simulink library "ChimeRouterLibBtc"  (R2022b)
settings: Solver=VariableStepAuto  StartTime=0.0  StopTime=10.0  RelTol=1e-3
libraries: TuneVar x3, FeaturePath x2, HandyTextFile x1, dspindex x1, RTC x1
settings Model: Creator=kl13806  LastModifiedBy=kl13806
settings SolverCC: AlgebraicLoopSolver=TrustRegion
settings DebuggingCC: UnconnectedInputMsg=warning  UnconnectedOutputMsg=warning  UnconnectedLineMsg=warning  SFMachineParentedDataDiag=warning
settings ModelReferenceCC: EnableRefExpFcnMdlSchedulingChecks=on
settings RTWCC: DLArmComputeVersion=19.05

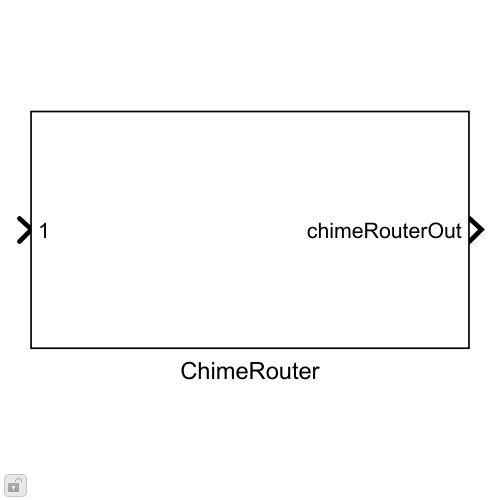
[thumbnail: Simulink's stored preview of the top-level diagram]
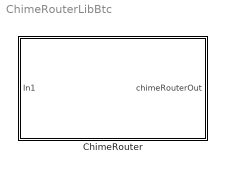
== system ChimeRouterLibBtc ==
  ChimeRouter : Subsystem  mask(Chimes ChimeRouter){Config=[]}
      mask prompts: Config "ChimeRouterConfig"
      mask init:
      | blkh=gcbh;
      | Config=BTConfig.Assert(blkh,Config);
      | 
      | Config.Validate();

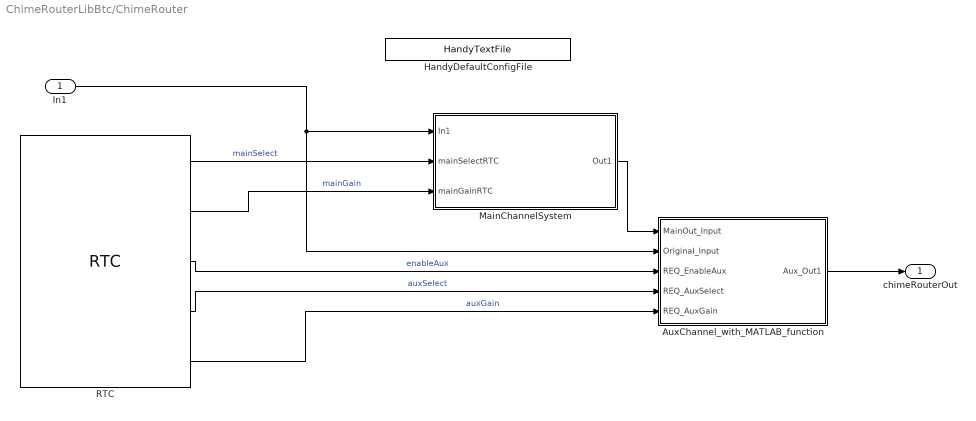
== system ChimeRouterLibBtc/ChimeRouter ==
  In1 : Inport
  AuxChannel_with_MATLAB_function : Subsystem
  HandyDefaultConfigFile : HandyTextFile/HandyTextFile  TemplateSource=Config  FileSuffix=Init  OpenDialogOnLoad=off  UseThisBlockName=off  AddGrandParentNamePrefix=off  TheDefaultText=|  ShowInLibBrowser=on
      | % $(FILENAME) Setup model parameters for each "Init" callback (e.g. update diagram)
      | sample_rate_in_hertz = 44100;
      | frame_size = 32;
      | sysin_channel_count = 2;
      settings: SourceProductName=Bose Talaria
  MainChannelSystem : Subsystem
  RTC : RTC/RTC  REQ_Priority=RTC_Mask.NormalPriority  RequestAtInit=off  EnableRequest=off  REQElemName1=MainSelect  REQElemType1=int32  REQElemWidth1=length(Config.MainSelect(:)')  REQElemInitial1=[]  REQElemName2=MainGain  REQElemType2=single  REQElemWidth2=length(Config.MainGain)  REQElemInitial2=[]  REQElemName3=EnableAux  REQElemType3=int32  REQElemWidth3=length(Config.EnableAux)  REQElemInitial3=[]  REQElemName4=AuxSelect  REQElemType4=int32  REQElemWidth4=length(Config.PAuxSelect)  REQElemInitial4=[]  REQElemName5=AuxGain  REQElemType5=single  REQElemWidth5=length(Config.PAuxGain)  REQElemInitial5=[]  REQElemType6=uint32  REQElemWidth6=1  REQElemInitial6=[]  REQElemType7=uint32  REQElemWidth7=1  REQElemInitial7=[]  REQElemType8=uint32  REQElemWidth8=1  REQElemInitial8=[]  REQElemType9=uint32  REQElemWidth9=1  REQElemInitial9=[]  REQElemType10=uint32  REQElemWidth10=1  REQElemInitial10=[]  EnableResponse=on  EnableRSP_StatusIn=off  RSPElemType1=uint32  RSPElemWidth1=1  RSPElemType2=uint32  RSPElemWidth2=1  RSPElemType3=uint32  RSPElemWidth3=1  RSPElemType4=uint32  RSPElemWidth4=1  RSPElemType5=uint32  RSPElemWidth5=1  RSPElemType6=uint32  RSPElemWidth6=1  RSPElemType7=uint32  RSPElemWidth7=1  RSPElemType8=uint32  RSPElemWidth8=1  RSPElemType9=uint32  RSPElemWidth9=1  RSPElemType10=uint32  RSPElemWidth10=1  EnableNotification=off  EnableNTF_PrepTrig=off  NTFElemType1=uint32  NTFElemWidth1=1  NTFElemType2=uint32  NTFElemWidth2=1  NTFElemType3=uint32  NTFElemWidth3=1  NTFElemType4=uint32  NTFElemWidth4=1  NTFElemType5=uint32  NTFElemWidth5=1  NTFElemType6=uint32  NTFElemWidth6=1  NTFElemType7=uint32  NTFElemWidth7=1  NTFElemType8=uint32  NTFElemWidth8=1  NTFElemType9=uint32  NTFElemWidth9=1  NTFElemType10=uint32  NTFElemWidth10=1  MaskMessageName=Set
      settings: SourceProductName=Bose Talaria
  chimeRouterOut : Outport  VectorParamsAs1DForOutWhenUnconnected=off
  wires:
  MainChannelSystem/1(Out1) -> AuxChannel_with_MATLAB_function/1(MainOut_Input)
  AuxChannel_with_MATLAB_function/1(Aux_Out1) -> chimeRouterOut/1
  In1/1 -> AuxChannel_with_MATLAB_function/2(Original_Input), MainChannelSystem/1(In1)
  RTC/3 -> AuxChannel_with_MATLAB_function/3(REQ_EnableAux)  "enableAux"
  RTC/4 -> AuxChannel_with_MATLAB_function/4(REQ_AuxSelect)  "auxSelect"
  RTC/5 -> AuxChannel_with_MATLAB_function/5(REQ_AuxGain)  "auxGain"
  RTC/1 -> MainChannelSystem/2(mainSelectRTC)  "mainSelect"
  RTC/2 -> MainChannelSystem/3(mainGainRTC)  "mainGain"

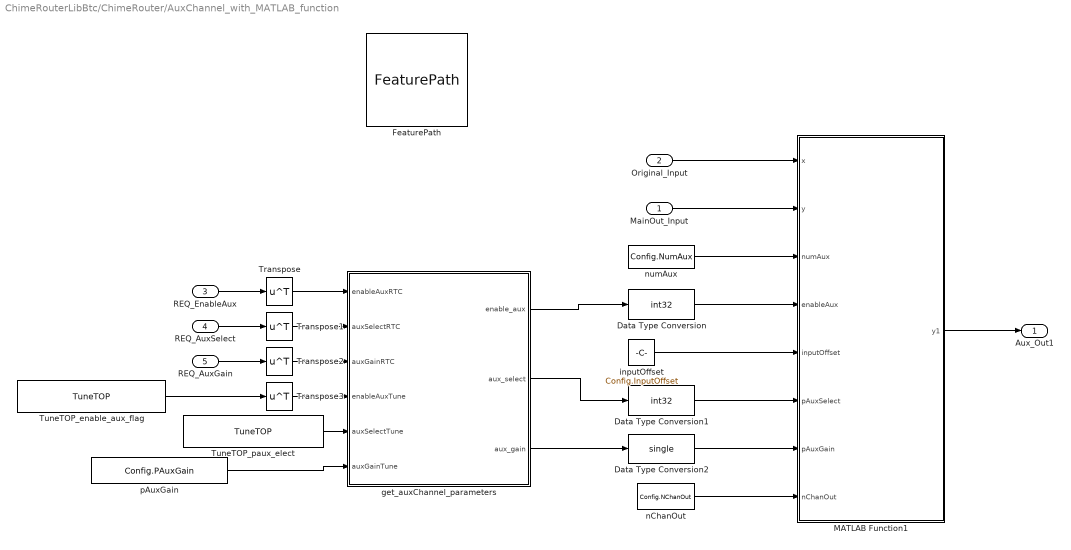
== system ChimeRouterLibBtc/ChimeRouter/AuxChannel_with_MATLAB_function ==
  MainOut_Input : Inport  PortDimensions=[Config.FrameSize Config.NChanOut]
  Original_Input : Inport  Port=2
  REQ_EnableAux : Inport  Port=3
  REQ_AuxSelect : Inport  Port=4
  REQ_AuxGain : Inport  Port=5
  Data Type Conversion : DataTypeConversion  OutDataTypeStr=int32  SaturateOnIntegerOverflow=off  RndMeth=Floor
  Data Type Conversion1 : DataTypeConversion  OutDataTypeStr=int32  SaturateOnIntegerOverflow=off  RndMeth=Floor
  Data Type Conversion2 : DataTypeConversion  OutDataTypeStr=single  SaturateOnIntegerOverflow=off  RndMeth=Floor
  FeaturePath : FeaturePath/FeaturePath  FeatureName=ASDRouterAuxChannel  IsGroup=on  GroupNumber=-1  IsModule=off  TriggerInit=[450 -186 565 -79]
      settings: SourceProductName=Bose Talaria
  MATLAB Function1 : MATLAB Function  TreatAsAtomicUnit=on
  Transpose{,1..3} (4 alike) : Math  Operator=transpose  SignedPower=on
  TuneTOP_enable_aux_flag : TuneVar/TuneTOP  TriggerInit=[50 212 220 248]  TopName=tune_top_enable_aux  TuneName=tune_top_enable_aux  DataType=int32  TunabilityNumber=1  MinValue=[]  MaxValue=[]  BankNumber=0  PreOverlay=false  PostOverlay=false  UseSameName=on  MaskValue=Config.EnableAux
      settings: SourceProductName=Bose Talaria
  TuneTOP_paux_elect : TuneVar/TuneTOP  TriggerInit=[240 252 400 288]  TopName=tune_top_paux_select  TuneName=tune_top_paux_select  DataType=int32  TunabilityNumber=1  MinValue=[]  MaxValue=[]  BankNumber=0  PreOverlay=false  PostOverlay=false  UseSameName=on  MaskValue=Config.PAuxSelect
      settings: SourceProductName=Bose Talaria
  get_auxChannel_parameters : MATLAB Function  TreatAsAtomicUnit=on
  inputOffset : Constant  Value=Config.InputOffset  OutDataTypeStr=int32
  nChanOut : Constant  Value=Config.NChanOut  OutDataTypeStr=int32
  numAux : Constant  Value=Config.NumAux  OutDataTypeStr=int32
  pAuxGain : Constant  Value=Config.PAuxGain  VectorParams1D=off  OutDataTypeStr=single
  Aux_Out1 : Outport  PortDimensions=[Config.FrameSize Config.NChanOut]  VectorParamsAs1DForOutWhenUnconnected=off
  wires:
  nChanOut/1 -> MATLAB Function1/8(nChanOut)
  REQ_EnableAux/1 -> Transpose/1
  TuneTOP_paux_elect/1 -> get_auxChannel_parameters/5(auxSelectTune)
  Transpose/1 -> get_auxChannel_parameters/1(enableAuxRTC)
  Transpose2/1 -> get_auxChannel_parameters/3(auxGainRTC)
  TuneTOP_enable_aux_flag/1 -> Transpose3/1
  inputOffset/1 -> MATLAB Function1/5(inputOffset)
  MainOut_Input/1 -> MATLAB Function1/2(y)
  MATLAB Function1/1(y1) -> Aux_Out1/1
  get_auxChannel_parameters/1(enable_aux) -> Data Type Conversion/1
  Transpose1/1 -> get_auxChannel_parameters/2(auxSelectRTC)
  REQ_AuxGain/1 -> Transpose2/1
  get_auxChannel_parameters/2(aux_select) -> Data Type Conversion1/1
  Data Type Conversion2/1 -> MATLAB Function1/7(pAuxGain)
  Original_Input/1 -> MATLAB Function1/1(x)
  Data Type Conversion/1 -> MATLAB Function1/4(enableAux)
  REQ_AuxSelect/1 -> Transpose1/1
  Data Type Conversion1/1 -> MATLAB Function1/6(pAuxSelect)
  pAuxGain/1 -> get_auxChannel_parameters/6(auxGainTune)
  Transpose3/1 -> get_auxChannel_parameters/4(enableAuxTune)
  numAux/1 -> MATLAB Function1/3(numAux)
  get_auxChannel_parameters/3(aux_gain) -> Data Type Conversion2/1

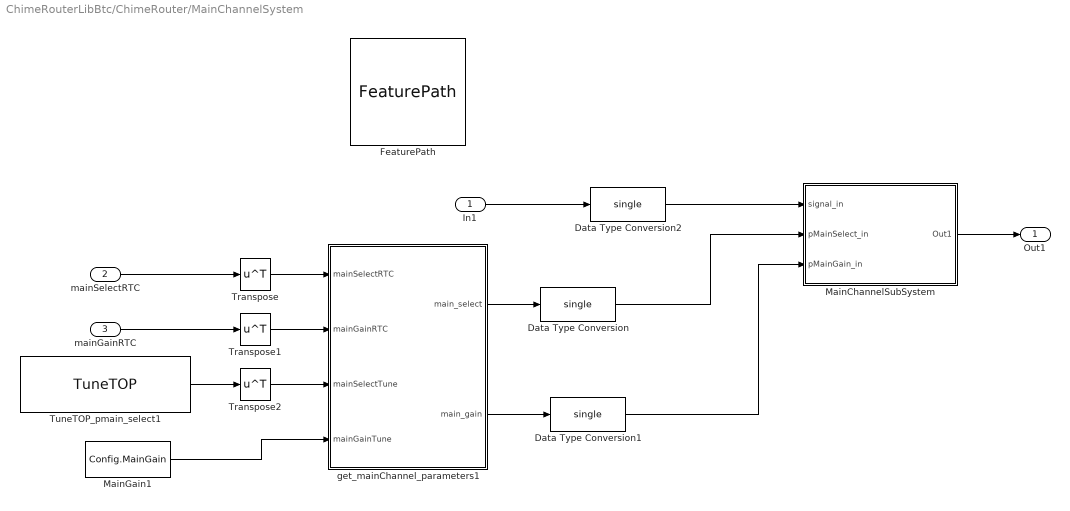
== system ChimeRouterLibBtc/ChimeRouter/MainChannelSystem ==
  In1 : Inport
  mainSelectRTC : Inport  Port=2
  mainGainRTC : Inport  Port=3
  Data Type Conversion : DataTypeConversion  OutDataTypeStr=single  SaturateOnIntegerOverflow=off  RndMeth=Floor
  Data Type Conversion1 : DataTypeConversion  OutDataTypeStr=single  SaturateOnIntegerOverflow=off  RndMeth=Floor
  Data Type Conversion2 : DataTypeConversion  OutDataTypeStr=single  SaturateOnIntegerOverflow=off  RndMeth=Floor
  FeaturePath : FeaturePath/FeaturePath  FeatureName=ASDRouterMainChannel  IsGroup=on  GroupNumber=-1  IsModule=off  TriggerInit=[-175 -121 -60 -14]
      settings: SourceProductName=Bose Talaria
  MainChannelSubSystem : Subsystem  TreatAsAtomicUnit=on
  MainGain1 : Constant  Value=Config.MainGain  VectorParams1D=off  OutDataTypeStr=single
  Transpose : Math  Operator=transpose  SignedPower=on
  Transpose1 : Math  Operator=transpose  SignedPower=on
  Transpose2 : Math  Operator=transpose  SignedPower=on
  TuneTOP_pmain_select1 : TuneVar/TuneTOP  TriggerInit=[-505 197 -335 253]  TopName=tune_top_main_select  TuneName=tune_top_main_select  DataType=single  TunabilityNumber=1  MinValue=[]  MaxValue=[]  BankNumber=0  PreOverlay=false  PostOverlay=false  UseSameName=on  MaskValue=Config.MainSelect
      settings: SourceProductName=Bose Talaria
  get_mainChannel_parameters1 : MATLAB Function  TreatAsAtomicUnit=on
  Out1 : Outport  PortDimensions=[Config.FrameSize Config.NChanOut]  VectorParamsAs1DForOutWhenUnconnected=off
  wires:
  In1/1 -> Data Type Conversion2/1
  MainChannelSubSystem/1(Out1) -> Out1/1
  TuneTOP_pmain_select1/1 -> Transpose2/1
  Transpose2/1 -> get_mainChannel_parameters1/3(mainSelectTune)
  Data Type Conversion1/1 -> MainChannelSubSystem/3(pMainGain_in)
  mainGainRTC/1 -> Transpose1/1
  Transpose/1 -> get_mainChannel_parameters1/1(mainSelectRTC)
  Data Type Conversion/1 -> MainChannelSubSystem/2(pMainSelect_in)
  get_mainChannel_parameters1/2(main_gain) -> Data Type Conversion1/1
  Transpose1/1 -> get_mainChannel_parameters1/2(mainGainRTC)
  mainSelectRTC/1 -> Transpose/1
  MainGain1/1 -> get_mainChannel_parameters1/4(mainGainTune)
  get_mainChannel_parameters1/1(main_select) -> Data Type Conversion/1
  Data Type Conversion2/1 -> MainChannelSubSystem/1(signal_in)

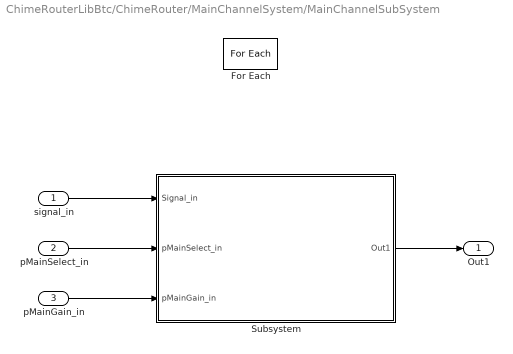
== system ChimeRouterLibBtc/ChimeRouter/MainChannelSystem/MainChannelSubSystem ==
  signal_in : Inport
  pMainSelect_in : Inport  Port=2  Partition=on  PartitionDimension=2  PartitionWidth=1  PartitionOffset=0
  pMainGain_in : Inport  Port=3  Partition=on  PartitionDimension=2  PartitionWidth=1  PartitionOffset=0
  For Each : ForEach  DisableCoverage=on
  Subsystem : Subsystem
  Out1 : Outport  ConcatenationDimension=2  VectorParamsAs1DForOutWhenUnconnected=off
  wires:
  pMainGain_in/1 -> Subsystem/3(pMainGain_in)
  pMainSelect_in/1 -> Subsystem/2(pMainSelect_in)
  signal_in/1 -> Subsystem/1(Signal_in)
  Subsystem/1(Out1) -> Out1/1

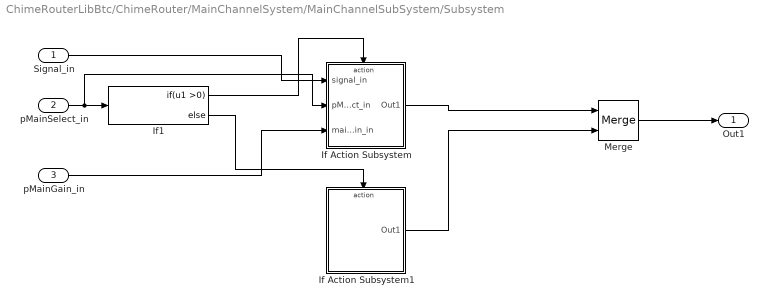
== system ChimeRouterLibBtc/ChimeRouter/MainChannelSystem/MainChannelSubSystem/Subsystem ==
  Signal_in : Inport
  pMainSelect_in : Inport  Port=2
  pMainGain_in : Inport  Port=3
  If Action Subsystem : Subsystem  TreatAsAtomicUnit=on
  If Action Subsystem1 : Subsystem  TreatAsAtomicUnit=on
  If1 : If  IfExpression=u1 >0
  Merge : Merge
  Out1 : Outport  VectorParamsAs1DForOutWhenUnconnected=off
  wires:
  If1/2 -> If Action Subsystem1/Action
  Merge/1 -> Out1/1
  If Action Subsystem1/1(Out1) -> Merge/2
  If Action Subsystem/1(Out1) -> Merge/1
  pMainGain_in/1 -> If Action Subsystem/3(mainGain_in)
  Signal_in/1 -> If Action Subsystem/1(signal_in)
  If1/1 -> If Action Subsystem/Action
  pMainSelect_in/1 -> If1/1, If Action Subsystem/2(pMainSelect_in)

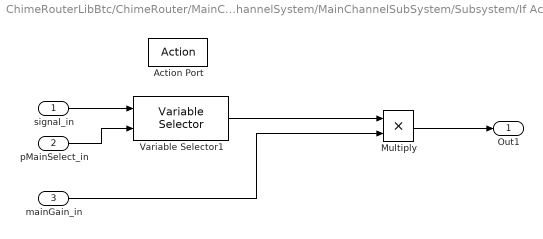
== system ChimeRouterLibBtc/ChimeRouter/MainChannelSystem/MainChannelSubSystem/Subsystem/If Action Subsystem ==
  signal_in : Inport
  pMainSelect_in : Inport  Port=2
  mainGain_in : Inport  Port=3
  Action Port : ActionPort
  Multiply : Product
  Variable Selector1 : dspindex/Variable Selector  NumInputs=1  rowsOrCols=Columns  IdxMode=Variable  Elements=tempSelect  ZerOneIdxMode=One-based  errmode=Clip Index  FillMode=on  FillValues=0
  Out1 : Outport  VectorParamsAs1DForOutWhenUnconnected=off
  wires:
  pMainSelect_in/1 -> Variable Selector1/2
  signal_in/1 -> Variable Selector1/1
  Variable Selector1/1 -> Multiply/1
  Multiply/1 -> Out1/1
  mainGain_in/1 -> Multiply/2

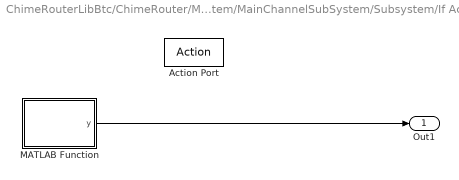
== system ChimeRouterLibBtc/ChimeRouter/MainChannelSystem/MainChannelSubSystem/Subsystem/If Action Subsystem1 ==
  Action Port : ActionPort
  MATLAB Function : MATLAB Function  TreatAsAtomicUnit=on
  Out1 : Outport  VectorParamsAs1DForOutWhenUnconnected=off
  wires:
  MATLAB Function/1(y) -> Out1/1

== matlab function ChimeRouterLibBtc/ChimeRouter/AuxChannel_with_MATLAB_function/MATLAB Function1 ==
  data: x input; y1 output; y input; numAux input; enableAux input; inputOffset input; pAuxSelect input; pAuxGain input; nChanOut input
function y1 = fcn(x, y, numAux, enableAux, inputOffset, pAuxSelect, pAuxGain, nChanOut)
%tempSelect=zeros(1,nChanOut*length(numAux));
%tempGain=ones(1,nChanOut*length(numAux));
for i=1:length(numAux)
   if(enableAux(i))
     tempSelect = inputOffset + pAuxSelect((i-1)*nChanOut+1:i*nChanOut);   %Account for Matlab 1 index
     tempGain = pAuxGain((i-1)*nChanOut+1:i*nChanOut);   %Account for Matlab 1 index
     for(ch=1:nChanOut)
       if (tempSelect(ch) > inputOffset)
            y(:,ch)=y(:,ch) + x(:, tempSelect(ch)) * tempGain(ch);
       end
     end
   end
   inputOffset = inputOffset + numAux(i);
end
y1 = y;

== matlab function ChimeRouterLibBtc/ChimeRouter/AuxChannel_with_MATLAB_function/get_auxChannel_parameters ==
  data: enableAuxRTC input; enable_aux output; auxSelectRTC input; auxGainRTC input; enableAuxTune input; auxSelectTune input; auxGainTune input; aux_select output; aux_gain output
function [enable_aux, aux_select, aux_gain] = get_auxChannel_parameters(...
    enableAuxRTC, auxSelectRTC, auxGainRTC,... % RTC message parameters
    enableAuxTune,auxSelectTune, auxGainTune) % Tune parameters

    Numiters=length(auxSelectRTC);
    aux_select=zeros(1,Numiters);
    aux_gain=zeros(1,Numiters);    
    enable_aux=zeros(size(enableAuxRTC));  
    enable_aux = double(enableAuxTune);   
    aux_select = double(auxSelectTune);
    aux_gain = double(auxGainTune); % Set to auxGainTune if a default is to be set

    for auxind=1:(Numiters)
        
    %if (auxSelectRTC(auxind))
        aux_select(auxind) = (auxSelectRTC(auxind));       
    %end  
    %if (auxGainRTC(auxind))
        aux_gain(auxind) = (auxGainRTC(auxind));       
    %end
    end
    enable_aux=double(enableAuxRTC);
%     for auxind=1:length(size(enableAuxRTC))
%     if(enableAuxRTC(auxind))
%             enable_aux(auxind)=enableAuxRTC(auxind);
%     end
%     end

== matlab function ChimeRouterLibBtc/ChimeRouter/MainChannelSystem/get_mainChannel_parameters1 ==
  data: mainSelectRTC input; main_select output; mainGainRTC input; mainSelectTune input; mainGainTune input; main_gain output
function [main_select, main_gain] = get_mainChannel_parameters(...
    mainSelectRTC, mainGainRTC,... % RTC message parameters
    mainSelectTune, mainGainTune) % Tune parameters

    % initialize to zeros
    Numiters=length(mainSelectRTC);
    main_select=zeros(1,Numiters);
    main_gain=zeros(1,Numiters);
    
    % convert data type
    main_select = double(mainSelectTune);
    main_gain = double(mainGainTune); % Set to mainSelectTune if a default is to be set
for mainind=1:(Numiters)
    if (mainSelectRTC(mainind))
        main_select(mainind) = (mainSelectRTC(mainind));       
    end  
    if (mainSelectRTC(mainind))
        main_gain(mainind) = (mainGainRTC(mainind));        
    end
end

== matlab function ChimeRouterLibBtc/ChimeRouter/MainChannelSystem/MainChannelSubSystem/Subsystem/If Action Subsystem1/MATLAB Function ==
  data: y output size=[L,1]; L parameter
function y = fcn(L)
% zeros
y = zeros(L,1);
